simulink model "modelLinearAna"  (R2017a)
settings: Solver=VariableStepAuto  StartTime=0.0  StopTime=10.0  RelTol=1e-3
values from neighbouring files (symbols this model uses):
  K = 1.098    [param.m]
  taux = 0.977    [param.m]
settings Model: Creator=arek  LastModifiedBy=arek

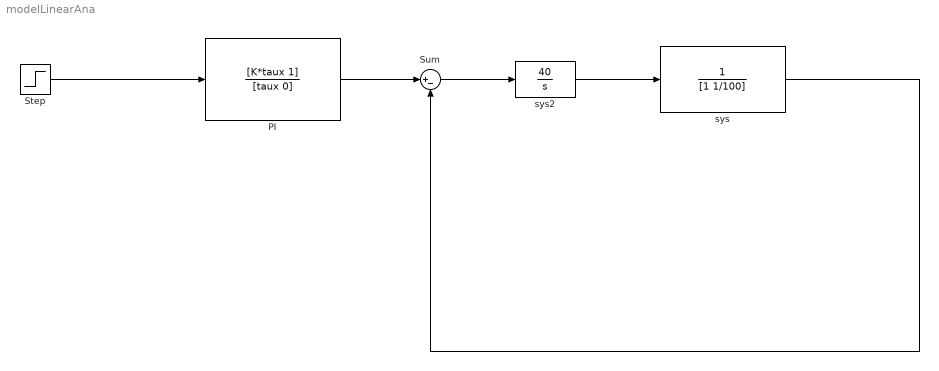
== system modelLinearAna ==
  PI : TransferFcn  Numerator=[K*taux 1]  Denominator=[taux 0]
  Step : Step  SampleTime=0
  Sum : Sum  Inputs=|+-
  sys : TransferFcn  Numerator=1  Denominator=[1 1/100]
  sys2 : TransferFcn  Numerator=40  Denominator=[1 0]
  wires:
  PI/1 -> Sum/1
  sys/1 -> Sum/2
  Sum/1 -> sys2/1
  sys2/1 -> sys/1
  Step/1 -> PI/1
